simulink library "tqd"  (R2021b)
settings: Solver=VariableStepAuto  StartTime=0.0  StopTime=10.0  RelTol=1e-3
undefined symbols (not defined in the file or in its folder): ATQD_APSDecReq_X_kph, ATQD_APSDecReq_Y_mps2, ATQD_APSDecReqCMD_X_kph, ATQD_APSDecReqTs_X_pct, ATQD_APSDecTimeGain_X_Deg, ATQD_APSDecTimeGain_Y_s, ATQD_APSReqLowSpd_X_Deg, ATQD_AutoHoldReleaseBPS_X_Deg, ATQD_AWDLoadTrqnsGain_X_kg, ATQD_AWDLoadTrqnsGain_Y_pct, ATQD_BOSEnBPSPosn_X_kph, ATQD_BOSMap_X_rpm, ATQD_BOSMap_Y_pct, ATQD_CreepBaseTqD_X_kph, ATQD_CreepBaseTqD_Y_Deg, ATQD_CreepBaseTqR_X_kph, ATQD_CreepBaseTqR_Y_Deg, ATQD_CreepBPSDisPosn_X_Deg, ATQD_CreepBPSDisPosnR_X_Deg, ATQD_CreepBPSEnPosn_X_Deg, ATQD_CreepBPSEnPosnR_X_Deg, ATQD_CreepDeltaTq_X_kph, ATQD_CreepIterm_X_kph, ATQD_CreepIterm_Y_kph, ATQD_CreepItermMaxLimit_X_pct, ATQD_CreepPreloadTime_X_kph, ATQD_CreepPreloadTq_X_kph, ATQD_CreepPreloadTq_Y_s, ATQD_CreepProtTq_X_Deg, ATQD_CreepPterm_X_kph, ATQD_CreepPterm_Y_kph, ATQD_ECOTqMapD_X_rpm, ATQD_ECOTqMapD_Y_pct, ATQD_EOPDTqMapDCon_X_rpm, ATQD_EOPDTqMapDCon_Y_Deg, ATQD_EstInitVehWeight_X_c, ATQD_LHMRollGenMapD_X_rpm, ATQD_LHMRollGenMapD_Y_rpm, ATQD_LHMTqMapD_X_rpm, ATQD_LHMTqMapD_Y_pct, ATQD_NL1TqMapD_X_rpm, ATQD_NL1TqMapD_Y_pct, ATQD_NOPDTqMapDCon_X_rpm, ATQD_NOPDTqMapDCon_Y_Deg, ATQD_NRMRrEDUSpRat_X_rpm, ATQD_NRMRrEDUSpRat_Y_Nm, ATQD_OPDHoldDownRelDelay_X_Deg, ATQD_OPDHoldEnSpd_X_Deg, ATQD_OPDHoldRelDetTime_X_Deg, ATQD_OPDHoldReleaseTq_X_Deg, ATQD_OrigPedTqLowLim_X_Deg, ATQD_OrigPedTqLowLim_Y_pct, ATQD_PedalMapClimbUpLim_X_rpm, ATQD_PedalMapClimbUpLim_Y_Deg, ATQD_PreLoadTq_X_s, ATQD_RollGenMapEL1_X_rpm, ATQD_RollGenMapEL1_Y_rpm, ATQD_SL1TqMapD_X_rpm, ATQD_SL1TqMapD_Y_pct, ATQD_SlideRegenTqGain_X_Gps ... (+491)
libraries: hcu_lib x83, simulink x73, tqr x1
(part 17 of 19)

== stateflow chart tqd/TQD/TorqueDemand/Signal_convert/SWC2_Subsystem/Speed Setting Mode/ACC Speed Setting ON/ACCSetSpd_241018 ==
  state MeterSpd
    state OFF_Error_Disable
      en:
      VTQD_ACCSetSpd_raw32 =  min(VTQD_ACCActiveMetSpdHi_raw32, VTQD_SpdLim4SetSpd_raw32);
      VTQD_ACCSetSpd_raw32 = max(VTQD_ACCActiveMetSpdLo_raw32, VTQD_ACCSetSpd_raw32);
      VTQD_ACCSavedSetSpd_raw32 = VTQD_ACCSetSpd_raw32;
      du:
      VTQD_ACCSetSpd_raw32 =  min(VTQD_ACCActiveMetSpdHi_raw32, VTQD_SpdLim4SetSpd_raw32);
      VTQD_ACCSetSpd_raw32 = max(VTQD_ACCActiveMetSpdLo_raw32, VTQD_ACCSetSpd_raw32);
      VTQD_ACCSavedSetSpd_raw32 = VTQD_ACCSetSpd_raw32;
    state Terminal
      %Do Nothing
    state Standby
      en:
      VTQD_ACCSetSpd_raw32 =  min(VTQD_ACCActiveMetSpdHi_raw32, VTQD_SpdLim4SetSpd_raw32);
      VTQD_ACCSetSpd_raw32 = max(VTQD_ACCActiveMetSpdLo_raw32, VTQD_ACCSetSpd_raw32);
      VTQD_ACCSavedSetSpd_raw32 = VTQD_ACCSetSpd_raw32;
      du:
      VTQD_ACCSetSpd_raw32 =  min(VTQD_ACCActiveMetSpdHi_raw32, VTQD_SpdLim4SetSpd_raw32);
      VTQD_ACCSetSpd_raw32 = max(VTQD_ACCActiveMetSpdLo_raw32, VTQD_ACCSetSpd_raw32);
      VTQD_ACCSavedSetSpd_raw32 = VTQD_ACCSetSpd_raw32;
    state Active_Override_ShutOff
      (default) -> (junction 749) : {VTQD_ACCSetSpd_raw32 = VTQD_ACCSavedSetSpd_raw32;}
      MeterSpd.Active_Override_ShutOff -> (junction 830) [order 1]
      (junction 830) -> (junction 834) [order 1] : [VTQD_DistanceUnit_flg == VINP_Distanceunit_flg || VTQD_ACCSavedSetSpd_raw32 <= ONE_FLOAT]
      (junction 834) -> (junction 749) : {VTQD_ACCSetSpd_raw32 = min(VTQD_ACCActiveMetSpdHi_raw32, VTQD_ACCSavedSetSpd_raw32);
          |  VTQD_ACCSavedSetSpd_raw32 = VTQD_ACCSetSpd_raw32;}
      (junction 749) -> (junction 751) [order 1] : [VINP_ADASACCSta_enum == ENUM_ADASACCSTA_ACTIVE]
      (junction 751) -> (junction 757) [order 1] : [VTQD_Set2MeterSpd_flg ||...
          |  VTQD_SetRoadSpdLim_flg]
      (junction 757) -> (junction 1115) [order 1] : [VTQD_Set2MeterSpd_flg]
      (junction 830) -> (junction 832) [order 2]
      (junction 837) -> (junction 834)
      (junction 749) -> (junction 798) [order 2]
      (junction 751) -> (junction 762) [order 2]
      (junction 757) -> (junction 759) [order 2] : {VTQD_ACCSetSpd_raw32 =  min(VTQD_ACCActiveMetSpdHi_raw32, VTQD_SpdLim4SetSpd_raw32);
          |  VTQD_ACCSetSpd_raw32 = max(VTQD_ACCActiveMetSpdLo_raw32, VTQD_ACCSetSpd_raw32);
          |  VTQD_ACCSavedSetSpd_raw32 = VTQD_ACCSetSpd_raw32;
          |  VTQD_DistanceUnit_flg = VINP_Distanceunit_flg;}
      (junction 1115) -> (junction 1114) : {VTQD_ACCSetSpd_raw32 =  min(VTQD_ACCActiveMetSpdHi_raw32, VVMC_MeterIndSpeed_raw32);
          |  VTQD_ACCSetSpd_raw32 = max(VTQD_ACCActiveMetSpdLo_raw32, VTQD_ACCSetSpd_raw32);
          |  VTQD_ACCSavedSetSpd_raw32 = VTQD_ACCSetSpd_raw32;
          |  VTQD_DistanceUnit_flg = VINP_Distanceunit_flg;}
      (junction 832) -> (junction 819) [order 1] : [VINP_Distanceunit_flg]
      (junction 832) -> (junction 833) [order 2] : {VTQD_ACCSavedSetSpd_raw32 = (VTQD_ACCSavedSetSpd_raw32 * MPH2KPH)}
      (junction 819) -> (junction 827) : {VTQD_ACCSavedSetSpd_raw32 = (VTQD_ACCSavedSetSpd_raw32 * KPH2MPH)}
      (junction 762) -> (junction 766) [order 1] : [(VTQD_SWC2ScrollUpSta_enum == ENUM_SWCBOTTONPRESS_SHORTPRESS ||...
          |   VTQD_SWC2ScrollDownSta_enum == ENUM_SWCBOTTONPRESS_SHORTPRESS) &&...
          |  !VVMC_LVDAACCStatusInformation_flg]
      (junction 766) -> (junction 771) [order 1] : [VTQD_SWC2ScrollUpSta_enum == ENUM_SWCBOTTONPRESS_SHORTPRESS]
      (junction 762) -> (junction 792) [order 2]
      (junction 766) -> (junction 779) [order 2] : {VTQD_ACCSetSpd_raw32 =  min(VTQD_ACCActiveMetSpdHi_raw32, VTQD_ACCSavedSetSpd_raw32 - ONE_FLOAT);
          |  VTQD_ACCSetSpd_raw32 = max(VTQD_ACCActiveMetSpdLo_raw32, VTQD_ACCSetSpd_raw32);
          |  VTQD_ACCSavedSetSpd_raw32 = VTQD_ACCSetSpd_raw32;
          |  VTQD_DistanceUnit_flg = VINP_Distanceunit_flg;}
      (junction 771) -> (junction 774) : {VTQD_ACCSetSpd_raw32 =  min(VTQD_ACCActiveMetSpdHi_raw32, VTQD_ACCSavedSetSpd_raw32 + ONE_FLOAT);
          |  VTQD_ACCSetSpd_raw32 = max(VTQD_ACCActiveMetSpdLo_raw32, VTQD_ACCSetSpd_raw32);
          |  VTQD_ACCSavedSetSpd_raw32 = VTQD_ACCSetSpd_raw32;
          |  VTQD_DistanceUnit_flg = VINP_Distanceunit_flg;}
      (junction 827) -> (junction 816) [order 1] : [VTQD_ACCSavedSetSpd_raw32 < KTQD_ACCActiveMetSpdLoMPH_mph]
      (junction 833) -> (junction 817) [order 1] : [VTQD_ACCSavedSetSpd_raw32 < KTQD_ACCActiveMetSpdLo_kph]
      (junction 816) -> (junction 820) : {VTQD_ACCSavedSetSpd_raw32 = KTQD_ACCActiveMetSpdLoMPH_mph}
      (junction 833) -> (junction 828) [order 2]
      (junction 817) -> (junction 815) : {VTQD_ACCSavedSetSpd_raw32 = KTQD_ACCActiveMetSpdLo_kph}
      (junction 827) -> (junction 818) [order 2]
      (junction 820) -> (junction 818)
      (junction 815) -> (junction 828)
      (junction 818) -> (junction 826)
      (junction 828) -> (junction 821)
      (junction 821) -> (junction 829) [order 1] : [VTQD_ACCSavedSetSpd_raw32 > KTQD_ACCActiveMetSpdHi_kph]
      (junction 826) -> (junction 822) [order 1] : [VTQD_ACCSavedSetSpd_raw32 > KTQD_ACCActiveMetSpdHiMPH_mph]
      (junction 821) -> (junction 823) [order 2]
      (junction 829) -> (junction 831) : {VTQD_ACCSavedSetSpd_raw32 = KTQD_ACCActiveMetSpdHi_kph}
      (junction 826) -> (junction 835) [order 2]
      (junction 822) -> (junction 824) : {VTQD_ACCSavedSetSpd_raw32 = KTQD_ACCActiveMetSpdHiMPH_mph}
      (junction 792) -> (junction 785) [order 1] : [(VTQD_SWC2ScrollUpSta_enum == ENUM_SWCBOTTONPRESS_LONGPRESS ||...
          |   VTQD_SWC2ScrollDownSta_enum == ENUM_SWCBOTTONPRESS_LONGPRESS) &&...
          |  !VVMC_LVDAACCStatusInformation_flg]
      (junction 785) -> (junction 790) [order 1] : [VTQD_SWC2ScrollUpSta_enum == ENUM_SWCBOTTONPRESS_LONGPRESS]
      (junction 831) -> (junction 823)
      (junction 824) -> (junction 835)
      (junction 792) -> (junction 809) [order 2] : {VTQD_ACCSetSpd_raw32 = VTQD_ACCSavedSetSpd_raw32;
          |  VTQD_ACCSavedSetSpd_raw32 = VTQD_ACCSetSpd_raw32;
          |  VTQD_DistanceUnit_flg = VINP_Distanceunit_flg;}
      (junction 785) -> (junction 793) [order 2] : {VTQD_ACCSetSpd_raw32 = max(VTQD_ACCActiveMetSpdLo_raw32, ceil(VTQD_ACCSavedSetSpd_raw32 / VTQD_SetSpdDeltaLong_raw32 - ONE_FLOAT) * VTQD_SetSpdDeltaLong_raw32);
          |  VTQD_ACCSetSpd_raw32 = min (VTQD_ACCActiveMetSpdHi_raw32, VTQD_ACCSetSpd_raw32);
          |  VTQD_ACCSavedSetSpd_raw32 = VTQD_ACCSetSpd_raw32;
          |  VTQD_DistanceUnit_flg = VINP_Distanceunit_flg;}
      (junction 790) -> (junction 783) : {VTQD_ACCSetSpd_raw32 = min(VTQD_ACCActiveMetSpdHi_raw32, floor(VTQD_ACCSavedSetSpd_raw32 / VTQD_SetSpdDeltaLong_raw32 + ONE_FLOAT) * VTQD_SetSpdDeltaLong_raw32);
          |  VTQD_ACCSetSpd_raw32 = max (VTQD_ACCActiveMetSpdLo_raw32, VTQD_ACCSetSpd_raw32);
          |  VTQD_ACCSavedSetSpd_raw32 = VTQD_ACCSetSpd_raw32;
          |  VTQD_DistanceUnit_flg = VINP_Distanceunit_flg;}
      (junction 823) -> (junction 825)
      (junction 835) -> (junction 836)
      (junction 825) -> (junction 836)
      (junction 836) -> (junction 837)
      (junction 798) -> (junction 806) [order 1] : [VINP_ADASACCSta_enum == ENUM_ADASACCSTA_OVERRIDE]
      (junction 806) -> (junction 804) [order 1] : [KTQD_ACCOVRDSpdAdj_flg &&...
          | (VTQD_Set2MeterSpd_flg ||...
          |  VTQD_SetRoadSpdLim_flg)]
      (junction 804) -> (junction 1119) [order 1] : [VTQD_Set2MeterSpd_flg]
      (junction 798) -> (junction 807) [order 2] : {VTQD_ACCSetSpd_raw32 = VTQD_ACCSavedSetSpd_raw32;
          |  VTQD_ACCSavedSetSpd_raw32 = VTQD_ACCSetSpd_raw32;
          |  VTQD_DistanceUnit_flg = VINP_Distanceunit_flg;}
      (junction 806) -> (junction 811) [order 2] : {VTQD_ACCSetSpd_raw32 = VTQD_ACCSavedSetSpd_raw32;
          |  VTQD_ACCSavedSetSpd_raw32 = VTQD_ACCSetSpd_raw32;
          |  VTQD_DistanceUnit_flg = VINP_Distanceunit_flg;}
      (junction 804) -> (junction 803) [order 2] : {VTQD_ACCSetSpd_raw32 =  min(VTQD_ACCActiveMetSpdHi_raw32, VTQD_SpdLim4SetSpd_raw32);
          |  VTQD_ACCSetSpd_raw32 = max(VTQD_ACCActiveMetSpdLo_raw32, VTQD_ACCSetSpd_raw32);
          |  VTQD_ACCSavedSetSpd_raw32 = VTQD_ACCSetSpd_raw32;
          |  VTQD_DistanceUnit_flg = VINP_Distanceunit_flg;}
      (junction 1119) -> (junction 1118) : {VTQD_ACCSetSpd_raw32 =  min(VTQD_ACCActiveMetSpdHi_raw32, VVMC_MeterIndSpeed_raw32);
          |  VTQD_ACCSetSpd_raw32 = max(VTQD_ACCActiveMetSpdLo_raw32, VTQD_ACCSetSpd_raw32);
          |  VTQD_ACCSavedSetSpd_raw32 = VTQD_ACCSetSpd_raw32;
          |  VTQD_DistanceUnit_flg = VINP_Distanceunit_flg;}
    (default) -> MeterSpd.OFF_Error_Disable [order 3]
    MeterSpd.Terminal -> MeterSpd.OFF_Error_Disable [order 2] : [VINP_ADASACCSta_enum ~= ENUM_ADASACCSTA_ACTIVE &&...
        |  VINP_ADASACCSta_enum ~= ENUM_ADASACCSTA_OVERRIDE &&...
        |  VINP_ADASACCSta_enum ~= ENUM_ADASACCSTA_SHUTOFF]
    MeterSpd.OFF_Error_Disable -> MeterSpd.Terminal [order 2] : [VINP_ADASACCSta_enum == ENUM_ADASACCSTA_ACTIVE ||...
        |  VINP_ADASACCSta_enum == ENUM_ADASACCSTA_OVERRIDE ||...
        |  VINP_ADASACCSta_enum == ENUM_ADASACCSTA_SHUTOFF]
    MeterSpd.Terminal -> MeterSpd.Active_Override_ShutOff [order 1] : [VINP_ADASACCSta_enum == ENUM_ADASACCSTA_ACTIVE ||...
        |  VINP_ADASACCSta_enum == ENUM_ADASACCSTA_OVERRIDE ||...
        |  VINP_ADASACCSta_enum == ENUM_ADASACCSTA_SHUTOFF]
    MeterSpd.Active_Override_ShutOff -> MeterSpd.Terminal [order 2] : [VINP_ADASACCSta_enum ~= ENUM_ADASACCSTA_ACTIVE &&...
        |  VINP_ADASACCSta_enum ~= ENUM_ADASACCSTA_OVERRIDE &&...
        |  VINP_ADASACCSta_enum ~= ENUM_ADASACCSTA_SHUTOFF]
    MeterSpd.OFF_Error_Disable -> MeterSpd.Standby [order 1] : [VINP_ADASACCSta_enum == ENUM_ADASACCSTA_STANDBY]
    MeterSpd.Standby -> MeterSpd.OFF_Error_Disable [order 2] : [VINP_ADASACCSta_enum ~= ENUM_ADASACCSTA_STANDBY]
    MeterSpd.Active_Override_ShutOff -> MeterSpd.Standby [order 1] : [VINP_ADASACCSta_enum == ENUM_ADASACCSTA_STANDBY]
    MeterSpd.Standby -> MeterSpd.Active_Override_ShutOff [order 1] : [VINP_ADASACCSta_enum == ENUM_ADASACCSTA_ACTIVE ||...
        |  VINP_ADASACCSta_enum == ENUM_ADASACCSTA_OVERRIDE ||...
        |  VINP_ADASACCSta_enum == ENUM_ADASACCSTA_SHUTOFF]
    (default) -> MeterSpd.Active_Override_ShutOff [order 2] : [VINP_ADASACCSta_enum == ENUM_ADASACCSTA_ACTIVE ||...
        |  VINP_ADASACCSta_enum == ENUM_ADASACCSTA_OVERRIDE ||...
        |  VINP_ADASACCSta_enum == ENUM_ADASACCSTA_SHUTOFF]
    (default) -> MeterSpd.Standby [order 1] : [VINP_ADASACCSta_enum == ENUM_ADASACCSTA_STANDBY]
  state RoadSpd
    state OFF_Error_Disable
      en:
      VTQD_ACCSetSpd_raw32 =  min(VTQD_ACCActiveMetSpdHi_raw32, VTQD_SpdLim4SetSpd_raw32);
      VTQD_ACCSetSpd_raw32 = max(VTQD_ACCActiveMetSpdLo_raw32, VTQD_ACCSetSpd_raw32);
      VTQD_ACCSavedSetSpd_raw32 = VTQD_ACCSetSpd_raw32;
      du:
      VTQD_ACCSetSpd_raw32 =  min(VTQD_ACCActiveMetSpdHi_raw32, VTQD_SpdLim4SetSpd_raw32);
      VTQD_ACCSetSpd_raw32 = max(VTQD_ACCActiveMetSpdLo_raw32, VTQD_ACCSetSpd_raw32);
      VTQD_ACCSavedSetSpd_raw32 = VTQD_ACCSetSpd_raw32;
    state Terminal
      %Do Nothing
    state Standby
      (default) -> (junction 987) : {VTQD_StandbyDisRoadSpd_flg = FALSE;}
      RoadSpd.Standby -> (junction 1029) [order 1]
      (junction 1029) -> (junction 1030) [order 1] : [VTQD_DistanceUnit_flg == VINP_Distanceunit_flg || VTQD_ACCSavedSetSpd_raw32 <= ONE_FLOAT]
      (junction 1030) -> (junction 987) : {VTQD_ACCSetSpd_raw32 = min(VTQD_ACCActiveMetSpdHi_raw32, VTQD_ACCSavedSetSpd_raw32);
          |  VTQD_ACCSavedSetSpd_raw32 = VTQD_ACCSetSpd_raw32;}
      (junction 987) -> (junction 1102) [order 1] : [VTQD_RoadSpdActive2Standby_flg &&...
          | (VTQD_StandbyDisRoadSpd_flg || !VTQD_ADASSLIFSpdLimDet_flg)]
      (junction 1029) -> (junction 1031) [order 2]
      (junction 1048) -> (junction 1030)
      (junction 987) -> (junction 1104) [order 2]
      (junction 1102) -> (junction 999)
      (junction 1031) -> (junction 1032) [order 1] : [VINP_Distanceunit_flg]
      (junction 1031) -> (junction 1034) [order 2] : {VTQD_ACCSavedSetSpd_raw32 = (VTQD_ACCSavedSetSpd_raw32 * MPH2KPH)}
      (junction 1032) -> (junction 1028) : {VTQD_ACCSavedSetSpd_raw32 = (VTQD_ACCSavedSetSpd_raw32 * KPH2MPH)}
      (junction 1104) -> (junction 999) [order 1] : [VTQD_SWC2ScrollUpSta_enum ~= ENUM_SWCBOTTONPRESS_NOPRESS ||...
          |  VTQD_SWC2ScrollDownSta_enum ~= ENUM_SWCBOTTONPRESS_NOPRESS ||...
          |  VTQD_StandbyDisRoadSpd_flg]
      (junction 999) -> (junction 1000) [order 1] : [VTQD_SWC2ScrollUpSta_enum == ENUM_SWCBOTTONPRESS_SHORTPRESS ||...
          |  VTQD_SWC2ScrollDownSta_enum == ENUM_SWCBOTTONPRESS_SHORTPRESS]
      (junction 1000) -> (junction 1001) [order 1] : [VTQD_SWC2ScrollUpSta_enum == ENUM_SWCBOTTONPRESS_SHORTPRESS]
      (junction 1104) -> (junction 991) [order 2] : {VTQD_ACCSetSpd_raw32 =  min(VTQD_ACCActiveMetSpdHi_raw32, VTQD_SpdLim4SetSpd_raw32);
          |  VTQD_ACCSetSpd_raw32 = max(VTQD_ACCActiveMetSpdLo_raw32, VTQD_ACCSetSpd_raw32);
          |  VTQD_ACCSavedSetSpd_raw32 = VTQD_ACCSetSpd_raw32;
          |  VTQD_DistanceUnit_flg = VINP_Distanceunit_flg;
          |  VTQD_RoadSpdActive2Standby_flg = FALSE;}
      (junction 999) -> (junction 1007) [order 2]
      (junction 1000) -> (junction 1005) [order 2] : {VTQD_ACCSetSpd_raw32 =  min(VTQD_ACCActiveMetSpdHi_raw32, VTQD_ACCSavedSetSpd_raw32 - ONE_FLOAT);
          |  VTQD_ACCSetSpd_raw32 = max(VTQD_ACCActiveMetSpdLo_raw32, VTQD_ACCSetSpd_raw32);
          |  VTQD_ACCSavedSetSpd_raw32 = VTQD_ACCSetSpd_raw32;
          |  VTQD_DistanceUnit_flg = VINP_Distanceunit_flg;
          |  VTQD_StandbyDisRoadSpd_flg = TRUE;}
      (junction 1001) -> (junction 1006) : {VTQD_ACCSetSpd_raw32 =  min(VTQD_ACCActiveMetSpdHi_raw32, VTQD_ACCSavedSetSpd_raw32 + ONE_FLOAT);
          |  VTQD_ACCSetSpd_raw32 = max(VTQD_ACCActiveMetSpdLo_raw32, VTQD_ACCSetSpd_raw32);
          |  VTQD_ACCSavedSetSpd_raw32 = VTQD_ACCSetSpd_raw32;
          |  VTQD_DistanceUnit_flg = VINP_Distanceunit_flg;
          |  VTQD_StandbyDisRoadSpd_flg = TRUE;}
      (junction 1028) -> (junction 1033) [order 1] : [VTQD_ACCSavedSetSpd_raw32 < KTQD_ACCActiveMetSpdLoMPH_mph]
      (junction 1034) -> (junction 1035) [order 1] : [VTQD_ACCSavedSetSpd_raw32 < KTQD_ACCActiveMetSpdLo_kph]
      (junction 1033) -> (junction 1043) : {VTQD_ACCSavedSetSpd_raw32 = KTQD_ACCActiveMetSpdLoMPH_mph}
      (junction 1034) -> (junction 1038) [order 2]
      (junction 1035) -> (junction 1039) : {VTQD_ACCSavedSetSpd_raw32 = KTQD_ACCActiveMetSpdLo_kph}
      (junction 1028) -> (junction 1045) [order 2]
      (junction 1043) -> (junction 1045)
      (junction 1039) -> (junction 1038)
      (junction 1045) -> (junction 1042)
      (junction 1038) -> (junction 1040)
      (junction 1040) -> (junction 1041) [order 1] : [VTQD_ACCSavedSetSpd_raw32 > KTQD_ACCActiveMetSpdHi_kph]
      (junction 1042) -> (junction 1044) [order 1] : [VTQD_ACCSavedSetSpd_raw32 > KTQD_ACCActiveMetSpdHiMPH_mph]
      (junction 1040) -> (junction 1053) [order 2]
      (junction 1041) -> (junction 1049) : {VTQD_ACCSavedSetSpd_raw32 = KTQD_ACCActiveMetSpdHi_kph}
      (junction 1042) -> (junction 1054) [order 2]
      (junction 1044) -> (junction 1047) : {VTQD_ACCSavedSetSpd_raw32 = KTQD_ACCActiveMetSpdHiMPH_mph}
      (junction 1007) -> (junction 1011) [order 1] : [VTQD_SWC2ScrollUpSta_enum == ENUM_SWCBOTTONPRESS_LONGPRESS ||...
          |  VTQD_SWC2ScrollDownSta_enum == ENUM_SWCBOTTONPRESS_LONGPRESS]
      (junction 1011) -> (junction 1009) [order 1] : [VTQD_SWC2ScrollUpSta_enum == ENUM_SWCBOTTONPRESS_LONGPRESS]
      (junction 1007) -> (junction 1012) [order 2]
      (junction 1011) -> (junction 1010) [order 2] : {VTQD_ACCSetSpd_raw32 = max(VTQD_ACCActiveMetSpdLo_raw32, ceil(VTQD_ACCSavedSetSpd_raw32 / VTQD_SetSpdDeltaLong_raw32 - ONE_FLOAT) * VTQD_SetSpdDeltaLong_raw32);
          |  VTQD_ACCSetSpd_raw32 = min (VTQD_ACCActiveMetSpdHi_raw32, VTQD_ACCSetSpd_raw32);
          |  VTQD_ACCSavedSetSpd_raw32 = VTQD_ACCSetSpd_raw32;
          |  VTQD_DistanceUnit_flg = VINP_Distanceunit_flg;
          |  VTQD_StandbyDisRoadSpd_flg = TRUE;}
      (junction 1009) -> (junction 1008) : {VTQD_ACCSetSpd_raw32 = min(VTQD_ACCActiveMetSpdHi_raw32, floor(VTQD_ACCSavedSetSpd_raw32 / VTQD_SetSpdDeltaLong_raw32 + ONE_FLOAT) * VTQD_SetSpdDeltaLong_raw32);
          |  VTQD_ACCSetSpd_raw32 = max (VTQD_ACCActiveMetSpdLo_raw32, VTQD_ACCSetSpd_raw32);
          |  VTQD_ACCSavedSetSpd_raw32 = VTQD_ACCSetSpd_raw32;
          |  VTQD_DistanceUnit_flg = VINP_Distanceunit_flg;
          |  VTQD_StandbyDisRoadSpd_flg = TRUE;}
      (junction 1049) -> (junction 1053)
      (junction 1047) -> (junction 1054)
      (junction 1053) -> (junction 1046)
      (junction 1054) -> (junction 1050)
      (junction 1046) -> (junction 1050)
      (junction 1050) -> (junction 1048)
      (junction 1012) -> (junction 1023) [order 1] : [VTQD_LScrollPressShort_flg &&...
          |  VTQD_ADASSLIFSpdLimDet_flg]
      (junction 1023) -> (junction 1026) : {VTQD_ACCSetSpd_raw32 =  min(VTQD_ACCActiveMetSpdHi_raw32, VTQD_SpdLim4SetSpd_raw32);
          |  VTQD_ACCSetSpd_raw32 = max(VTQD_ACCActiveMetSpdLo_raw32, VTQD_ACCSetSpd_raw32);
          |  VTQD_ACCSavedSetSpd_raw32 = VTQD_ACCSetSpd_raw32;
          |  VTQD_DistanceUnit_flg = VINP_Distanceunit_flg;
          |  VTQD_StandbyDisRoadSpd_flg = FALSE;
          |  VTQD_RoadSpdActive2Standby_flg = FALSE;}
      (junction 1012) -> (junction 1022) [order 2] : {VTQD_ACCSetSpd_raw32 =  VTQD_ACCSavedSetSpd_raw32;
          |  VTQD_ACCSavedSetSpd_raw32 = VTQD_ACCSetSpd_raw32;
          |  VTQD_DistanceUnit_flg = VINP_Distanceunit_flg;}
    state Active_Override_ShutOff
      (default) -> (junction 883) : {VTQD_ACCSetSpd_raw32 = VTQD_ACCSavedSetSpd_raw32;}
      RoadSpd.Active_Override_ShutOff -> (junction 881) [order 1]
      (junction 881) -> (junction 882) [order 1] : [VTQD_DistanceUnit_flg == VINP_Distanceunit_flg || VTQD_ACCSavedSetSpd_raw32 <= ONE_FLOAT]
      (junction 882) -> (junction 883) : {VTQD_ACCSetSpd_raw32 = min(VTQD_ACCActiveMetSpdHi_raw32, VTQD_ACCSavedSetSpd_raw32);
          |  VTQD_ACCSavedSetSpd_raw32 = VTQD_ACCSetSpd_raw32;}
      (junction 883) -> (junction 884) [order 1] : [VINP_ADASACCSta_enum == ENUM_ADASACCSTA_ACTIVE]
      (junction 884) -> (junction 885) [order 1] : [VTQD_Set2MeterSpd_flg ||...
          |  VTQD_SetRoadSpdLim_flg]
      (junction 885) -> (junction 1124) [order 1] : [VTQD_Set2MeterSpd_flg]
      (junction 881) -> (junction 886) [order 2]
      (junction 915) -> (junction 882)
      (junction 883) -> (junction 919) [order 2]
      (junction 884) -> (junction 889) [order 2]
      (junction 885) -> (junction 888) [order 2] : {VTQD_ACCSetSpd_raw32 =  min(VTQD_ACCActiveMetSpdHi_raw32, VTQD_SpdLim4SetSpd_raw32);
          |  VTQD_ACCSetSpd_raw32 = max(VTQD_ACCActiveMetSpdLo_raw32, VTQD_ACCSetSpd_raw32);
          |  VTQD_ACCSavedSetSpd_raw32 = VTQD_ACCSetSpd_raw32;
          |  VTQD_DistanceUnit_flg = VINP_Distanceunit_flg;}
      (junction 1124) -> (junction 1123) : {VTQD_ACCSetSpd_raw32 =  min(VTQD_ACCActiveMetSpdHi_raw32, VVMC_MeterIndSpeed_raw32);
          |  VTQD_ACCSetSpd_raw32 = max(VTQD_ACCActiveMetSpdLo_raw32, VTQD_ACCSetSpd_raw32);
          |  VTQD_ACCSavedSetSpd_raw32 = VTQD_ACCSetSpd_raw32;
          |  VTQD_DistanceUnit_flg = VINP_Distanceunit_flg;}
      (junction 886) -> (junction 887) [order 1] : [VINP_Distanceunit_flg]
      (junction 886) -> (junction 893) [order 2] : {VTQD_ACCSavedSetSpd_raw32 = (VTQD_ACCSavedSetSpd_raw32 * MPH2KPH)}
      (junction 887) -> (junction 895) : {VTQD_ACCSavedSetSpd_raw32 = (VTQD_ACCSavedSetSpd_raw32 * KPH2MPH)}
      (junction 889) -> (junction 890) [order 1] : [(VTQD_SWC2ScrollUpSta_enum == ENUM_SWCBOTTONPRESS_SHORTPRESS ||...
          |   VTQD_SWC2ScrollDownSta_enum == ENUM_SWCBOTTONPRESS_SHORTPRESS) &&...
          |  !VVMC_LVDAACCStatusInformation_flg]
      (junction 890) -> (junction 891) [order 1] : [VTQD_SWC2ScrollUpSta_enum == ENUM_SWCBOTTONPRESS_SHORTPRESS]
      (junction 889) -> (junction 906) [order 2]
      (junction 890) -> (junction 904) [order 2] : {VTQD_ACCSetSpd_raw32 =  min(VTQD_ACCActiveMetSpdHi_raw32, VTQD_ACCSavedSetSpd_raw32 - ONE_FLOAT);
          |  VTQD_ACCSetSpd_raw32 = max(VTQD_ACCActiveMetSpdLo_raw32, VTQD_ACCSetSpd_raw32);
          |  VTQD_ACCSavedSetSpd_raw32 = VTQD_ACCSetSpd_raw32;
          |  VTQD_DistanceUnit_flg = VINP_Distanceunit_flg;}
      (junction 891) -> (junction 905) : {VTQD_ACCSetSpd_raw32 =  min(VTQD_ACCActiveMetSpdHi_raw32, VTQD_ACCSavedSetSpd_raw32 + ONE_FLOAT);
          |  VTQD_ACCSetSpd_raw32 = max(VTQD_ACCActiveMetSpdLo_raw32, VTQD_ACCSetSpd_raw32);
          |  VTQD_ACCSavedSetSpd_raw32 = VTQD_ACCSetSpd_raw32;
          |  VTQD_DistanceUnit_flg = VINP_Distanceunit_flg;}
      (junction 895) -> (junction 892) [order 1] : [VTQD_ACCSavedSetSpd_raw32 < KTQD_ACCActiveMetSpdLoMPH_mph]
      (junction 893) -> (junction 894) [order 1] : [VTQD_ACCSavedSetSpd_raw32 < KTQD_ACCActiveMetSpdLo_kph]
      (junction 892) -> (junction 897) : {VTQD_ACCSavedSetSpd_raw32 = KTQD_ACCActiveMetSpdLoMPH_mph}
      (junction 893) -> (junction 898) [order 2]
      (junction 894) -> (junction 899) : {VTQD_ACCSavedSetSpd_raw32 = KTQD_ACCActiveMetSpdLo_kph}
      (junction 895) -> (junction 896) [order 2]
      (junction 897) -> (junction 896)
      (junction 899) -> (junction 898)
      (junction 896) -> (junction 902)
      (junction 898) -> (junction 900)
      (junction 900) -> (junction 901) [order 1] : [VTQD_ACCSavedSetSpd_raw32 > KTQD_ACCActiveMetSpdHi_kph]
      (junction 902) -> (junction 903) [order 1] : [VTQD_ACCSavedSetSpd_raw32 > KTQD_ACCActiveMetSpdHiMPH_mph]
      (junction 900) -> (junction 909) [order 2]
      (junction 901) -> (junction 910) : {VTQD_ACCSavedSetSpd_raw32 = KTQD_ACCActiveMetSpdHi_kph}
      (junction 902) -> (junction 911) [order 2]
      (junction 903) -> (junction 912) : {VTQD_ACCSavedSetSpd_raw32 = KTQD_ACCActiveMetSpdHiMPH_mph}
      (junction 906) -> (junction 907) [order 1] : [(VTQD_SWC2ScrollUpSta_enum == ENUM_SWCBOTTONPRESS_LONGPRESS ||...
          |   VTQD_SWC2ScrollDownSta_enum == ENUM_SWCBOTTONPRESS_LONGPRESS) &&...
          |  !VVMC_LVDAACCStatusInformation_flg]
      (junction 907) -> (junction 908) [order 1] : [VTQD_SWC2ScrollUpSta_enum == ENUM_SWCBOTTONPRESS_LONGPRESS]
      (junction 910) -> (junction 909)
      (junction 912) -> (junction 911)
      (junction 906) -> (junction 916) [order 2] : {VTQD_ACCSetSpd_raw32 = VTQD_ACCSavedSetSpd_raw32;
          |  VTQD_ACCSavedSetSpd_raw32 = VTQD_ACCSetSpd_raw32;
          |  VTQD_DistanceUnit_flg = VINP_Distanceunit_flg;}
      (junction 907) -> (junction 917) [order 2] : {VTQD_ACCSetSpd_raw32 = max(VTQD_ACCActiveMetSpdLo_raw32, ceil(VTQD_ACCSavedSetSpd_raw32 / VTQD_SetSpdDeltaLong_raw32 - ONE_FLOAT) * VTQD_SetSpdDeltaLong_raw32);
          |  VTQD_ACCSetSpd_raw32 = min (VTQD_ACCActiveMetSpdHi_raw32, VTQD_ACCSetSpd_raw32);
          |  VTQD_ACCSavedSetSpd_raw32 = VTQD_ACCSetSpd_raw32;
          |  VTQD_DistanceUnit_flg = VINP_Distanceunit_flg;}
      (junction 908) -> (junction 918) : {VTQD_ACCSetSpd_raw32 = min(VTQD_ACCActiveMetSpdHi_raw32, floor(VTQD_ACCSavedSetSpd_raw32 / VTQD_SetSpdDeltaLong_raw32 + ONE_FLOAT) * VTQD_SetSpdDeltaLong_raw32);
          |  VTQD_ACCSetSpd_raw32 = max (VTQD_ACCActiveMetSpdLo_raw32, VTQD_ACCSetSpd_raw32);
          |  VTQD_ACCSavedSetSpd_raw32 = VTQD_ACCSetSpd_raw32;
          |  VTQD_DistanceUnit_flg = VINP_Distanceunit_flg;}
      (junction 909) -> (junction 913)
      (junction 911) -> (junction 914)
      (junction 913) -> (junction 914)
      (junction 914) -> (junction 915)
      (junction 919) -> (junction 920) [order 1] : [VINP_ADASACCSta_enum == ENUM_ADASACCSTA_OVERRIDE]
      (junction 920) -> (junction 921) [order 1] : [KTQD_ACCOVRDSpdAdj_flg &&...
          | (VTQD_Set2MeterSpd_flg ||...
          |  VTQD_SetRoadSpdLim_flg)]
      (junction 921) -> (junction 1128) [order 1] : [VTQD_Set2MeterSpd_flg]
      (junction 919) -> (junction 924) [order 2] : {VTQD_ACCSetSpd_raw32 = VTQD_ACCSavedSetSpd_raw32;
          |  VTQD_ACCSavedSetSpd_raw32 = VTQD_ACCSetSpd_raw32;
          |  VTQD_DistanceUnit_flg = VINP_Distanceunit_flg;}
      (junction 920) -> (junction 922) [order 2] : {VTQD_ACCSetSpd_raw32 = VTQD_ACCSavedSetSpd_raw32;
          |  VTQD_ACCSavedSetSpd_raw32 = VTQD_ACCSetSpd_raw32;
          |  VTQD_DistanceUnit_flg = VINP_Distanceunit_flg;}
      (junction 921) -> (junction 923) [order 2] : {VTQD_ACCSetSpd_raw32 =  min(VTQD_ACCActiveMetSpdHi_raw32, VTQD_SpdLim4SetSpd_raw32);
          |  VTQD_ACCSetSpd_raw32 = max(VTQD_ACCActiveMetSpdLo_raw32, VTQD_ACCSetSpd_raw32);
          |  VTQD_ACCSavedSetSpd_raw32 = VTQD_ACCSetSpd_raw32;
          |  VTQD_DistanceUnit_flg = VINP_Distanceunit_flg;}
      (junction 1128) -> (junction 1127) : {VTQD_ACCSetSpd_raw32 =  min(VTQD_ACCActiveMetSpdHi_raw32, VVMC_MeterIndSpeed_raw32);
          |  VTQD_ACCSetSpd_raw32 = max(VTQD_ACCActiveMetSpdLo_raw32, VTQD_ACCSetSpd_raw32);
          |  VTQD_ACCSavedSetSpd_raw32 = VTQD_ACCSetSpd_raw32;
          |  VTQD_DistanceUnit_flg = VINP_Distanceunit_flg;}
    (default) -> RoadSpd.OFF_Error_Disable [order 3]
    RoadSpd.Terminal -> RoadSpd.OFF_Error_Disable [order 2] : [VINP_ADASACCSta_enum ~= ENUM_ADASACCSTA_ACTIVE &&...
        |  VINP_ADASACCSta_enum ~= ENUM_ADASACCSTA_OVERRIDE &&...
        |  VINP_ADASACCSta_enum ~= ENUM_ADASACCSTA_SHUTOFF]
    RoadSpd.OFF_Error_Disable -> RoadSpd.Terminal [order 2] : [VINP_ADASACCSta_enum == ENUM_ADASACCSTA_ACTIVE ||...
        |  VINP_ADASACCSta_enum == ENUM_ADASACCSTA_OVERRIDE ||...
        |  VINP_ADASACCSta_enum == ENUM_ADASACCSTA_SHUTOFF]
        | {VTQD_RoadSpdActive2Standby_flg = FALSE;}
    RoadSpd.Terminal -> RoadSpd.Active_Override_ShutOff [order 1] : [VINP_ADASACCSta_enum == ENUM_ADASACCSTA_ACTIVE ||...
        |  VINP_ADASACCSta_enum == ENUM_ADASACCSTA_OVERRIDE ||...
        |  VINP_ADASACCSta_enum == ENUM_ADASACCSTA_SHUTOFF]
    RoadSpd.Active_Override_ShutOff -> RoadSpd.Terminal [order 2] : [VINP_ADASACCSta_enum ~= ENUM_ADASACCSTA_ACTIVE &&...
        |  VINP_ADASACCSta_enum ~= ENUM_ADASACCSTA_OVERRIDE &&...
        |  VINP_ADASACCSta_enum ~= ENUM_ADASACCSTA_SHUTOFF]
    RoadSpd.OFF_Error_Disable -> RoadSpd.Standby [order 1] : [VINP_ADASACCSta_enum == ENUM_ADASACCSTA_STANDBY]
    RoadSpd.Standby -> RoadSpd.OFF_Error_Disable [order 2] : [VINP_ADASACCSta_enum ~= ENUM_ADASACCSTA_STANDBY]
        | {VTQD_RoadSpdActive2Standby_flg = FALSE;}
    RoadSpd.Active_Override_ShutOff -> RoadSpd.Standby [order 1] : [VINP_ADASACCSta_enum == ENUM_ADASACCSTA_STANDBY]
        | {VTQD_RoadSpdActive2Standby_flg = TRUE;}
    RoadSpd.Standby -> RoadSpd.Active_Override_ShutOff [order 1] : [VINP_ADASACCSta_enum == ENUM_ADASACCSTA_ACTIVE ||...
        |  VINP_ADASACCSta_enum == ENUM_ADASACCSTA_OVERRIDE ||...
        |  VINP_ADASACCSta_enum == ENUM_ADASACCSTA_SHUTOFF]
        | {VTQD_RoadSpdActive2Standby_flg = FALSE;}
    (default) -> RoadSpd.Active_Override_ShutOff [order 2] : [VINP_ADASACCSta_enum == ENUM_ADASACCSTA_ACTIVE ||...
        |  VINP_ADASACCSta_enum == ENUM_ADASACCSTA_OVERRIDE ||...
        |  VINP_ADASACCSta_enum == ENUM_ADASACCSTA_SHUTOFF]
    (default) -> RoadSpd.Standby [order 1] : [VINP_ADASACCSta_enum == ENUM_ADASACCSTA_STANDBY]
  (default) -> MeterSpd : {VTQD_ACCSavedSetSpd_raw32 = ZERO_FLOAT;
      |  VTQD_RoadSpdActive2Standby_flg = FALSE;
      |  VTQD_StandbyDisRoadSpd_flg = FALSE}
  RoadSpd -> MeterSpd : [!VINP_IVIACCAdaptiveSta_flg]
  MeterSpd -> RoadSpd : [VINP_IVIACCAdaptiveSta_flg]
  data: VINP_ADASACCSta_enum input; ENUM_ADASACCSTA_SHUTOFF parameter; ENUM_ADASACCSTA_STANDBY parameter; ENUM_ADASACCSTA_OVERRIDE parameter; ENUM_ADASACCSTA_ACTIVE parameter; ZERO_FLOAT parameter; VTQD_ACCSetSpd_raw32 output single; VINP_IVIACCAdaptiveSta_flg input; VTQD_SpdLim4SetSpd_raw32 input; VTQD_ACCActiveMetSpdHi_raw32 input; VTQD_ACCActiveMetSpdLo_raw32 input; VTQD_Set2MeterSpd_flg input; VTQD_SWC2ScrollUpSta_enum input; VTQD_SWC2ScrollDownSta_enum input; ENUM_SWCBOTTONPRESS_SHORTPRESS parameter; ONE_FLOAT parameter; ENUM_SWCBOTTONPRESS_LONGPRESS parameter; VTQD_ACCSavedSetSpd_raw32 local single; VTQD_SetSpdDeltaLong_raw32 input; VTQD_SetRoadSpdLim_flg input; KTQD_ACCOVRDSpdAdj_flg parameter; KPH2MPH parameter; VTQD_DistanceUnit_flg local boolean; MPH2KPH parameter; KTQD_ACCActiveMetSpdHiMPH_mph parameter; KTQD_ACCActiveMetSpdHi_kph parameter; KTQD_ACCActiveMetSpdLoMPH_mph parameter; KTQD_ACCActiveMetSpdLo_kph parameter; VTQD_RoadSpdActive2Standby_flg local boolean; VINP_Distanceunit_flg input; VTQD_ADASSLIFSpdLimDet_flg input; VTQD_StandbyDisRoadSpd_flg local boolean; VTQD_LScrollPressShort_flg input; FALSE parameter; TRUE parameter; ENUM_SWCBOTTONPRESS_NOPRESS parameter; VVMC_LVDAACCStatusInformation_flg input; VVMC_MeterIndSpeed_raw32 input

== stateflow chart tqd/TQD/TorqueDemand/Signal_convert/SWC_Subsystem/Speed Control Mode ==
  state OFF
    en:
    VTQD_SpdCtrlMode_enum = ENUM_SPDCTRLMODE_OFF;
    VTQD_SpdCtrlSta_flg = FALSE;
  state ACC
    en:
    VTQD_SpdCtrlMode_enum = ENUM_SPDCTRLMODE_ACC;
    VTQD_SpdCtrlSta_flg = TRUE;
  state CC
    en:
    VTQD_SpdCtrlMode_enum = ENUM_SPDCTRLMODE_CC;
    VTQD_SpdCtrlSta_flg = TRUE;
  state MSA
    en:
    VTQD_SpdCtrlMode_enum = ENUM_SPDCTRLMODE_MSA;
    VTQD_SpdCtrlSta_flg = TRUE;
  state ISA
    en:
    VTQD_SpdCtrlMode_enum = ENUM_SPDCTRLMODE_ISA;
    VTQD_SpdCtrlSta_flg = TRUE;
  (default) -> OFF
  OFF -> (junction 29) [order 2]
  (junction 29) -> (junction 31) : [
      | VPMM_PowerSta_enum == ENUM_POWERSTA_READY &&...
      | VTQD_ShiftGearPosn_enum == ENUM_GEARPOSNTOCAN_D &&...
      | VINP_ADASACCSta_enum != ENUM_ADASACCSTA_OFF &&...
      | VTQD_SpdCtrlShortP_flg]
  (junction 26) -> (junction 93)
  (junction 100) -> (junction 26)
  (junction 40) -> OFF
  (junction 93) -> (junction 40)
  (junction 38) -> (junction 40)
  (junction 36) -> (junction 93)
  OFF -> ACC [order 1] : [
      | VPMM_PowerSta_enum == ENUM_POWERSTA_READY &&...
      | VTQD_ShiftGearPosn_enum == ENUM_GEARPOSNTOCAN_D &&...
      | VINP_ADASACCSta_enum == ENUM_ADASACCSTA_OFF && ...
      | VTQD_SpdCtrlShortP_flg
      | ]
  ACC -> (junction 38) [order 1] : [
      | VPMM_PowerSta_enum != ENUM_POWERSTA_READY ||...
      | VTQD_ShiftGearPosn_enum != ENUM_GEARPOSNTOCAN_D ||...
      | (VINP_ADASACCSta_enum == ENUM_ADASACCSTA_DISABLE ||...
      | VINP_ADASACCSta_enum == ENUM_ADASACCSTA_ERROR) ||...
      | VTQD_SpdCtrlLongP_flg
      | ]
  ACC -> CC [order 2] : [VTQD_SpdCtrlShortP_flg]
  CC -> (junction 36) [order 1] : [
      | VPMM_PowerSta_enum != ENUM_POWERSTA_READY||...
      | VTQD_ShiftGearPosn_enum != ENUM_GEARPOSNTOCAN_D ||...
      | VTQD_SpdCtrlLongP_flg
      | ]
  (junction 31) -> CC
  CC -> (junction 11) [order 2]
  (junction 11) -> (junction 14) [order 2]
  (junction 11) -> MSA [order 1] : [
      | VTQD_SpdCtrlShortP_flg && ...
      | (VINP_ADASISASta_enum == ENUM_ADASISASTA_DISABLE ||...
      | VINP_ADASISASta_enum == ENUM_ADASISASTA_ERROR || ...
      | !VTQD_IVIISAOffsetSpdCHOOSE_flg)
      | %add20230704
      | ]
  (junction 14) -> ISA : [
      | VTQD_SpdCtrlShortP_flg && ...
      | VINP_ADASISASta_enum == ENUM_ADASISASTA_OFF  && ...
      | VTQD_IVIISAOffsetSpdCHOOSE_flg
      | %add20230704
      | ]
  MSA -> ISA [order 2] : [
      | VINP_ADASISASta_enum == ENUM_ADASISASTA_OFF  && ...
      | VTQD_IVIISAOffsetSpdCHOOSE_flg
      | ]
  ISA -> (junction 100) [order 2] : [
      | VINP_ADASISASta_enum == ENUM_ADASISASTA_ERROR || ...
      | VINP_ADASISASta_enum == ENUM_ADASISASTA_DISABLE || ...
      | !VTQD_IVIISAOffsetSpdCHOOSE_flg
      | ]
  (junction 24) -> (junction 100)
  MSA -> (junction 19) [order 1]
  ISA -> (junction 21) [order 1]
  (junction 19) -> (junction 21)
  (junction 21) -> (junction 24) : [VPMM_PowerSta_enum != ENUM_POWERSTA_READY || ...
      | VTQD_ShiftGearPosn_enum != ENUM_GEARPOSNTOCAN_D ||...
      | VTQD_SpdCtrlShortP_flg || ...
      | VTQD_SpdCtrlLongP_flg
      | ]
  data: VPMM_PowerSta_enum input; VTQD_SpdCtrlShortP_flg input; VTQD_SpdCtrlLongP_flg input; ENUM_SPDCTRLMODE_OFF parameter; ENUM_SPDCTRLMODE_ACC parameter; ENUM_SPDCTRLMODE_CC parameter; ENUM_SPDCTRLMODE_ISA parameter; ENUM_SPDCTRLMODE_MSA parameter; FALSE parameter; ENUM_ADASACCSTA_DISABLE parameter; VINP_ADASACCSta_enum input; ENUM_POWERSTA_READY parameter; VINP_ADASISASta_enum input; ENUM_ADASISASTA_DISABLE parameter; VTQD_SpdCtrlMode_enum output uint8; VTQD_SpdCtrlSta_flg output boolean; TRUE parameter; VTQD_IVIISAOffsetSpdCHOOSE_flg input; ENUM_ADASISASTA_ERROR parameter; ENUM_ADASISASTA_OFF parameter; ENUM_ADASACCSTA_ERROR parameter; ENUM_ADASACCSTA_OFF parameter; VTQD_ShiftGearPosn_enum input; ENUM_GEARPOSNTOCAN_D parameter

== stateflow chart tqd/TQD/TorqueDemand/Signal_convert/SWC2_Subsystem/Speed Setting Mode/ACC Speed Setting ON/ACCSetSpd_Chart_W ==
  state ACCSetSpeed_W
    (default) -> (junction 431) : {VTQD_ACCSetSpd_kph = KTQD_ACCActiveMetSpdLo_raw32;
        |  VTQD_ACCSavedSetSpd_kph = KTQD_ACCActiveMetSpdLo_raw32;
        |  VTQD_UpDownDetCount_sec = ZERO_FLOAT;
        |  VTQD_StandbyOvrdDetEnd_flg = FALSE;}
        | %add20240904
    ACCSetSpeed_W -> (junction 538) [order 3]
    (junction 538) -> (junction 552) [order 1] : [VTQD_DistanceUnit_flg == VINP_Distanceunit_flg || VTQD_ACCSavedSetSpd_kph <= ONE_FLOAT]
    (junction 552) -> (junction 431) : {VTQD_ACCSetSpd_kph = min(KTQD_ACCActiveMetSpdHi_raw32, VTQD_ACCSavedSetSpd_kph);
        |  VTQD_ACCSavedSetSpd_kph = VTQD_ACCSetSpd_kph;}
        | %add20240918
    (junction 538) -> (junction 540) [order 2]
    (junction 550) -> (junction 552)
    (junction 431) -> (junction 432) : {VSCP_ActiveDown_flg = FALSE;
        |  VTQD_ActiveUp_flg = FALSE;
        |  VTQD_UpDownTimeCount_sec = ZERO_FLOAT;}
    (junction 540) -> (junction 542) [order 1] : [VINP_Distanceunit_flg == TRUE]
    (junction 540) -> (junction 636) [order 2] : {VTQD_ACCSavedSetSpd_kph = (VTQD_ACCSavedSetSpd_kph * MPH2KPH)}
    (junction 542) -> (junction 599) : {VTQD_ACCSavedSetSpd_kph = (VTQD_ACCSavedSetSpd_kph * KPH2MPH)}
    (junction 432) -> (junction 530) [order 1] : [VINP_ADASACCSta_enum == ENUM_ADASACCSTA_STANDBY ||...
        |  VINP_ADASACCSta_enum == ENUM_ADASACCSTA_OVERRIDE]
    (junction 530) -> (junction 433) [order 1] : [VTQD_SWC2SetDownSta_flg ||...
        |  VTQD_SWC2ResUpSta_flg]
        | %add20250825
    (junction 433) -> (junction 419) [order 1] : [VTQD_SWC2SetDownSta_flg == TRUE &&...
        |  VTQD_StandbyOvrdDetEnd_flg == FALSE &&...
        |  VTQD_AllowSetSpd_flg == TRUE]
    (junction 432) -> (junction 403) [order 2]
    (junction 530) -> (junction 533) [order 2] : {VTQD_StandbyOvrdDetEnd_flg = FALSE;
        |  VTQD_ACCSetSpd_kph = VTQD_ACCSavedSetSpd_kph;
        |  VTQD_ACCSavedSetSpd_kph = VTQD_ACCSetSpd_kph;
        |  VTQD_DistanceUnit_flg = VINP_Distanceunit_flg;}
    (junction 433) -> (junction 490) [order 2]
    (junction 419) -> (junction 408) : {VTQD_UpDownDetCount_sec = VTQD_UpDownDetCount_sec + task_time_s;}
    (junction 599) -> (junction 602) [order 1] : [VTQD_ACCSavedSetSpd_kph < KTQD_ACCActiveMetSpdLoMPH_mph]
    (junction 636) -> (junction 623) [order 1] : [VTQD_ACCSavedSetSpd_kph < KTQD_ACCActiveMetSpdLo_kph]
    (junction 602) -> (junction 604) : {VTQD_ACCSavedSetSpd_kph = KTQD_ACCActiveMetSpdLoMPH_mph}
    (junction 636) -> (junction 633) [order 2]
    (junction 623) -> (junction 619) : {VTQD_ACCSavedSetSpd_kph = KTQD_ACCActiveMetSpdLo_kph}
    (junction 599) -> (junction 606) [order 2]
    (junction 604) -> (junction 606)
    (junction 619) -> (junction 633)
    (junction 606) -> (junction 613)
    (junction 633) -> (junction 630)
    (junction 630) -> (junction 625) [order 1] : [VTQD_ACCSavedSetSpd_kph > KTQD_ACCActiveMetSpdHi_kph]
    (junction 613) -> (junction 608) [order 1] : [VTQD_ACCSavedSetSpd_kph > KTQD_ACCActiveMetSpdHiMPH_mph]
    (junction 403) -> (junction 395) [order 1] : [ (VTQD_SWC2SetDownSta_flg || ...
        |   VTQD_SWC2ResUpSta_flg) &&...
        |  (VTQD_StandbyOvrdDetEnd_flg == TRUE ||...
        |   VTQD_HoldResDet_flg == TRUE)]
        | %add20240906
    (junction 490) -> (junction 492) [order 1] : [VINP_ADASACCSta_enum == ENUM_ADASACCSTA_STANDBY &&...
        |  VTQD_SWC2ResUpSta_flg &&...
        |  VTQD_ACCSavedSetSpd_kph > ZERO_FLOAT]
        | %add20240825
    (junction 408) -> (junction 409) [order 1] : [VTQD_UpDownDetCount_sec > ZERO_FLOAT]
    (junction 409) -> (junction 405) [order 1] : [KTQD_ACCActiveMetSpdHi_raw32 >= VVMC_MeterIndSpeed_raw32 &&...
        |  VVMC_MeterIndSpeed_raw32 >= KTQD_ACCActiveMetSpdLo_raw32]
    (junction 630) -> (junction 632) [order 2]
    (junction 625) -> (junction 628) : {VTQD_ACCSavedSetSpd_kph = KTQD_ACCActiveMetSpdHi_kph}
    (junction 613) -> (junction 615) [order 2]
    (junction 608) -> (junction 612) : {VTQD_ACCSavedSetSpd_kph = KTQD_ACCActiveMetSpdHiMPH_mph}
    (junction 403) -> (junction 396) [order 2] : {VTQD_StandbyOvrdDetEnd_flg = FALSE;
        |  VTQD_HoldResDet_flg = FALSE;}
    (junction 395) -> (junction 399) : {VTQD_StandbyOvrdDetEnd_flg = TRUE;
        |  VTQD_HoldResDet_flg = TRUE;}
        | %add20240906
    (junction 490) -> (junction 496) [order 2]
    (junction 492) -> (junction 494) : {VTQD_StandbyOvrdDetEnd_flg = TRUE}
    (junction 408) -> (junction 436) [order 2] : {VTQD_ACCSetSpd_kph = VTQD_ACCSavedSetSpd_kph;
        |  VTQD_ACCSavedSetSpd_kph = VTQD_ACCSetSpd_kph;
        |  VTQD_DistanceUnit_flg = VINP_Distanceunit_flg;}
    (junction 409) -> (junction 410) [order 2]
    (junction 405) -> (junction 435) : {VTQD_ACCSetSpd_kph = VVMC_MeterIndSpeed_raw32;
        |  VTQD_ACCSavedSetSpd_kph = VTQD_ACCSetSpd_kph;
        |  VTQD_StandbyOvrdDetEnd_flg = TRUE;
        |  VTQD_UpDownDetCount_sec = ZERO_FLOAT;
        |  VTQD_DistanceUnit_flg = VINP_Distanceunit_flg;}
    (junction 628) -> (junction 632)
    (junction 612) -> (junction 615)
    (junction 632) -> (junction 547)
    (junction 615) -> (junction 544)
    (junction 547) -> (junction 544)
    (junction 544) -> (junction 550)
    (junction 494) -> (junction 496)
    (junction 410) -> (junction 429) [order 1] : [KTQD_ACCActiveMetSpdHi_raw32 < VVMC_MeterIndSpeed_raw32]
    (junction 496) -> (junction 407) : {VTQD_ACCSetSpd_kph = VTQD_ACCSavedSetSpd_kph;
        | VTQD_ACCSetSpd_kph = min ( KTQD_ACCActiveMetSpdHi_raw32, VTQD_ACCSetSpd_kph);
        | VTQD_ACCSetSpd_kph = max ( KTQD_ACCActiveMetSpdLo_raw32, VTQD_ACCSetSpd_kph);
        |  VTQD_ACCSavedSetSpd_kph = VTQD_ACCSetSpd_kph;
        |  VTQD_DistanceUnit_flg = VINP_Distanceunit_flg;}
        | %add20240907
    (junction 410) -> (junction 420) [order 2] : {VTQD_ACCSetSpd_kph = KTQD_ACCActiveMetSpdLo_raw32;
        |  VTQD_ACCSavedSetSpd_kph = VTQD_ACCSetSpd_kph;
        |  VTQD_StandbyOvrdDetEnd_flg = TRUE;
        |  VTQD_UpDownDetCount_sec = ZERO_FLOAT;
        |  VTQD_DistanceUnit_flg = VINP_Distanceunit_flg;}
    (junction 429) -> (junction 430) : {VTQD_ACCSetSpd_kph = KTQD_ACCActiveMetSpdHi_raw32;
        |  VTQD_ACCSavedSetSpd_kph = VTQD_ACCSetSpd_kph;
        |  VTQD_StandbyOvrdDetEnd_flg = TRUE;
        |  VTQD_UpDownDetCount_sec = ZERO_FLOAT;
        |  VTQD_DistanceUnit_flg = VINP_Distanceunit_flg;}
    (junction 399) -> (junction 396)
    (junction 396) -> (junction 438)
    (junction 438) -> (junction 417) [order 1] : [VINP_ADASACCSta_enum == ENUM_ADASACCSTA_ACTIVE]
    (junction 417) -> (junction 434) [order 1] : [VTQD_SWC2ScrollDownSta_enum == ENUM_SWCBOTTONPRESS_SHORTPRESS &&...
        |  VTQD_StandbyOvrdDetEnd_flg == FALSE &&...
        |  VVMC_LVDAACCStatusInformation_flg == FALSE]
        | %add20240825
    (junction 438) -> (junction 427) [order 2]
    (junction 417) -> (junction 653) [order 2]
    (junction 434) -> (junction 411) : {VTQD_UpDownDetCount_sec = VTQD_UpDownDetCount_sec + task_time_s;}
    (junction 653) -> (junction 655) [order 1] : [VTQD_SWC2SetDownSta_flg]
    (junction 411) -> (junction 437) [order 1] : [VTQD_UpDownDetCount_sec > ZERO_FLOAT]
    (junction 655) -> (junction 656) : {VTQD_ACCSetSpd_kph = max ( VVMC_MeterIndSpeed_raw32, KTQD_ACCActiveMetSpdLo_raw32);
        | VTQD_ACCSetSpd_kph = min ( KTQD_ACCActiveMetSpdHi_raw32, VTQD_ACCSetSpd_kph);
        |  VTQD_ACCSavedSetSpd_kph = VTQD_ACCSetSpd_kph;
        |  VTQD_DistanceUnit_flg = VINP_Distanceunit_flg}
        | %add20240907
    (junction 653) -> (junction 412) [order 2]
    (junction 411) -> (junction 406) [order 2] : {VTQD_ACCSetSpd_kph = VTQD_ACCSavedSetSpd_kph;
        |  VTQD_ACCSavedSetSpd_kph = VTQD_ACCSetSpd_kph;
        |  VTQD_DistanceUnit_flg = VINP_Distanceunit_flg;}
    (junction 437) -> (junction 428) : {VTQD_ACCSetSpd_kph = max(KTQD_ACCActiveMetSpdLo_raw32, VTQD_ACCSavedSetSpd_kph - ONE_FLOAT);
        | VTQD_ACCSetSpd_kph = min ( KTQD_ACCActiveMetSpdHi_raw32, VTQD_ACCSetSpd_kph);
        |  VTQD_ACCSavedSetSpd_kph = VTQD_ACCSetSpd_kph;
        |  VSCP_ActiveDown_flg = TRUE;
        |  VTQD_UpDownDetCount_sec = ZERO_FLOAT;
        |  VTQD_UpDownTimeCount_sec = task_time_s;
        |  VTQD_DistanceUnit_flg = VINP_Distanceunit_flg;}
        | %add20240907
    (junction 427) -> (junction 404) [order 1] : [VINP_ADASACCSta_enum == ENUM_ADASACCSTA_OFF ||...
        |  VINP_ADASACCSta_enum == ENUM_ADASACCSTA_DISABLE||...
        |  VINP_ADASACCSta_enum == ENUM_ADASACCSTA_ERROR]
    (junction 412) -> (junction 510) [order 1] : [VTQD_SWC2ScrollUpSta_enum == ENUM_SWCBOTTONPRESS_SHORTPRESS]
        | %add20240825
    (junction 510) -> (junction 413) [order 1] : [VTQD_StandbyOvrdDetEnd_flg == FALSE &&...
        |  VVMC_LVDAACCStatusInformation_flg == FALSE &&...
        |  VTQD_HoldResDet_flg == FALSE && ...
        | !VTQD_SWC2ResUpSta_flg]
        | %add20240905
    (junction 427) -> (junction 422) [order 2] : {VTQD_ACCSetSpd_kph = VTQD_ACCSavedSetSpd_kph;
        |  VTQD_ACCSavedSetSpd_kph = VTQD_ACCSetSpd_kph;
        |  VTQD_DistanceUnit_flg = VINP_Distanceunit_flg;}
    (junction 404) -> (junction 426) : {VTQD_ACCSetSpd_kph = KTQD_ACCActiveMetSpdLo_raw32;
        |  VTQD_ACCSavedSetSpd_kph = VTQD_ACCSetSpd_kph;
        |  VTQD_DistanceUnit_flg = VINP_Distanceunit_flg;}
        | %add20240905
    (junction 412) -> (junction 522) [order 2]
    (junction 510) -> (junction 512) [order 2]
    (junction 413) -> (junction 421) : {VTQD_ACCSetSpd_kph = min(KTQD_ACCActiveMetSpdHi_raw32, VTQD_ACCSavedSetSpd_kph + ONE_FLOAT);
        | VTQD_ACCSetSpd_kph = max(KTQD_ACCActiveMetSpdLo_raw32, VTQD_ACCSetSpd_kph);
        |  VTQD_ACCSavedSetSpd_kph = VTQD_ACCSetSpd_kph;
        |  VTQD_ActiveUp_flg = TRUE;
        |  VTQD_DistanceUnit_flg = VINP_Distanceunit_flg;}
        | %add20240825
    (junction 512) -> (junction 514) [order 1] : [VTQD_StandbyOvrdDetEnd_flg == FALSE &&...
        |  VVMC_LVDAACCStatusInformation_flg != FALSE]
    (junction 512) -> (junction 519) [order 2]
    (junction 514) -> (junction 516) : {VTQD_HoldResDet_flg = TRUE}
    (junction 519) -> (junction 522)
    (junction 516) -> (junction 519)
    (junction 522) -> (junction 416) : {VTQD_ACCSetSpd_kph = VTQD_ACCSavedSetSpd_kph;
        |  VTQD_ACCSavedSetSpd_kph = VTQD_ACCSetSpd_kph;
        |  VTQD_DistanceUnit_flg = VINP_Distanceunit_flg;}
    ACCSetSpeed_W -> (junction 568) [order 1] : [VINP_ADASACCSta_enum == ENUM_ADASACCSTA_ACTIVE &&...
        |  VTQD_SWC2ScrollDownSta_enum == ENUM_SWCBOTTONPRESS_LONGPRESS]
        | %add20240905
    (junction 568) -> (junction 556) [order 1] : [VTQD_DistanceUnit_flg == VINP_Distanceunit_flg]
    (junction 556) -> (junction 423)
    (junction 568) -> (junction 558) [order 2]
    (junction 560) -> (junction 556)
    (junction 423) -> (junction 466)
    (junction 558) -> (junction 566) [order 1] : [VINP_Distanceunit_flg == TRUE]
    (junction 558) -> (junction 571) [order 2] : {VTQD_ACCSavedSetSpd_kph = (VTQD_ACCSavedSetSpd_kph * MPH2KPH)}
    (junction 566) -> (junction 557) : {VTQD_ACCSavedSetSpd_kph = (VTQD_ACCSavedSetSpd_kph * KPH2MPH)}
    (junction 466) -> (junction 478) : {VTQD_ACCSetSpd_kph = max(KTQD_ACCActiveMetSpdLo_raw32, ceil(VTQD_ACCSavedSetSpd_kph / KTQD_SetSpdDeltaLong_kph - ONE_FLOAT) * KTQD_SetSpdDeltaLong_kph);
        | VTQD_ACCSetSpd_kph = min ( KTQD_ACCActiveMetSpdHi_raw32, VTQD_ACCSetSpd_kph);
        |  VTQD_ACCSavedSetSpd_kph = VTQD_ACCSetSpd_kph;
        |  VTQD_DistanceUnit_flg = VINP_Distanceunit_flg;}
        | %add20240907
    (junction 571) -> (junction 557)
    (junction 557) -> (junction 560)
    ACCSetSpeed_W -> (junction 585) [order 2] : [ VINP_ADASACCSta_enum == ENUM_ADASACCSTA_ACTIVE &&...
        |  VTQD_SWC2ScrollUpSta_enum == ENUM_SWCBOTTONPRESS_LONGPRESS]
        | %add20240905
    (junction 585) -> (junction 583) [order 1] : [VTQD_DistanceUnit_flg == VINP_Distanceunit_flg]
    (junction 583) -> (junction 479)
    (junction 585) -> (junction 584) [order 2]
    (junction 580) -> (junction 583)
    (junction 479) -> (junction 463)
    (junction 584) -> (junction 576) [order 1] : [VINP_Distanceunit_flg == TRUE]
    (junction 584) -> (junction 573) [order 2] : {VTQD_ACCSavedSetSpd_kph = (VTQD_ACCSavedSetSpd_kph * MPH2KPH)}
    (junction 576) -> (junction 582) : {VTQD_ACCSavedSetSpd_kph = (VTQD_ACCSavedSetSpd_kph * KPH2MPH)}
    (junction 463) -> (junction 461) : {VTQD_ACCSetSpd_kph = min(KTQD_ACCActiveMetSpdHi_raw32, floor(VTQD_ACCSavedSetSpd_kph / KTQD_SetSpdDeltaLong_kph + ONE_FLOAT) * KTQD_SetSpdDeltaLong_kph);
        | VTQD_ACCSetSpd_kph = max ( KTQD_ACCActiveMetSpdLo_raw32, VTQD_ACCSetSpd_kph);
        |  VTQD_ACCSavedSetSpd_kph = VTQD_ACCSetSpd_kph;
        |  VTQD_DistanceUnit_flg = VINP_Distanceunit_flg;}
        |  %add20240907
    (junction 573) -> (junction 582)
    (junction 582) -> (junction 580)
  data: VINP_ADASACCSta_enum input uint8; VTQD_SWC2ResUpSta_flg input boolean; VTQD_SWC2SetDownSta_flg input boolean; VVMC_MeterIndSpeed_raw32 input single; KTQD_ACCActiveMetSpdHi_raw32 input uint8; VINP_Distanceunit_flg input boolean; KTQD_ACCActiveMetSpdLo_raw32 input uint8; VTQD_ACCSetSpd_kph output single; KTQD_SetSpdDeltaLong_kph input uint8; VTQD_ACCSavedSetSpd_kph local single; ENUM_ADASACCSTA_STANDBY parameter uint8; ZERO_FLOAT parameter single; TRUE parameter boolean; ENUM_ADASACCSTA_ACTIVE parameter uint8; ONE_FLOAT parameter single; FALSE parameter boolean; VSCP_ActiveDown_flg local boolean; VTQD_UpDownTimeCount_sec local single; VTQD_ActiveUp_flg local boolean; VTQD_UpDownDetCount_sec local single; ENUM_ADASACCSTA_OVERRIDE parameter uint8; VTQD_StandbyOvrdDetEnd_flg local boolean; ENUM_ADASACCSTA_DISABLE parameter; ENUM_ADASACCSTA_OFF parameter; ENUM_ADASACCSTA_ERROR parameter; VVMC_LVDAACCStatusInformation_flg input; VTQD_HoldResDet_flg local boolean; VTQD_AllowSetSpd_flg input; task_time_s input; VTQD_DistanceUnit_flg local boolean; KPH2MPH parameter; MPH2KPH parameter; KTQD_ACCActiveMetSpdLo_kph parameter; KTQD_ACCActiveMetSpdLoMPH_mph parameter; KTQD_ACCActiveMetSpdHiMPH_mph parameter; KTQD_ACCActiveMetSpdHi_kph parameter; VTQD_SWC2ScrollUpSta_enum input; VTQD_SWC2ScrollDownSta_enum input; ENUM_SWCBOTTONPRESS_LONGPRESS parameter; ENUM_SWCBOTTONPRESS_SHORTPRESS parameter
